simulink model "Flight_Controllers_PIL"  (R2024a)
settings: Solver=FixedStepAuto  StartTime=0.0  StopTime=tFinal  FixedStep=0.02  RelTol=1e-3  EnableMultiTasking=on
values from neighbouring files (symbols this model uses):
  bOmega = -bThrust/mThrust    (= 168.963839792)    [Load_VehicleParams.m]
  Cant_cosine_Loss = cos(fanCantAngle)    [Load_VehicleParams.m]
  g = 9.807    [Load_VehicleParams.m]
  g_Offset = 5/6    (= 0.833333333333)    [Load_VehicleParams.m]
  Kd_LatPos = 0    [Load_Controller_Gains_14.m]
  Kd_LatVel = 0    [Load_Controller_Gains_14.m]
  Kd_Pitch = 41.5    [Load_Controller_Gains_14.m]
  Ki_LatPos = 0    [Load_Controller_Gains_14.m]
  Ki_LatVel = 0    [Load_Controller_Gains_14.m]
  Ki_Pitch = 0.65    [Load_Controller_Gains_14.m]
  Kp_LatPos = 0.4    [Load_Controller_Gains_14.m]
  Kp_LatVel = -0.3    [Load_Controller_Gains_14.m]
  Kp_Pitch = 16    [Load_Controller_Gains_14.m]
  mOmega = 1/mThrust    (= 1.62153397114)    [Load_VehicleParams.m]
  N_LatPos = 0    [Load_Controller_Gains_14.m]
  N_LatVel = 0    [Load_Controller_Gains_14.m]
  N_Pitch = 85.6    [Load_Controller_Gains_14.m]
  nFans = 4    [Load_VehicleParams.m]
  pitch_Cmd_Limit = 7*pi/180    (= 0.12217304764)    [Load_Controller_Gains_14.m]
  T = 0.02    [run_Lander_GNC_Sim.m]
  tau_vCmd = 0.1    [Load_Controller_Gains_14.m]
  Ts_Control = 1/50    (= 0.02)    [run_Lander_GNC_Sim.m]
  velCmd_Limit = 7*pi/180    (= 0.12217304764)    [Load_Controller_Gains_14.m]
undefined symbols (not defined in the file or in its folder): den_Gc_z_Pitch, den_Gc_z_Pos, DiscIntNeverNeededParam, num_Gc_z_Pitch, num_Gc_z_Pos, posCntrl_Integr_Limit, tau_LatPos, tau_xCmd, vCmd_Integr_Limit
libraries: slpidlib x17
(part 2 of 3)

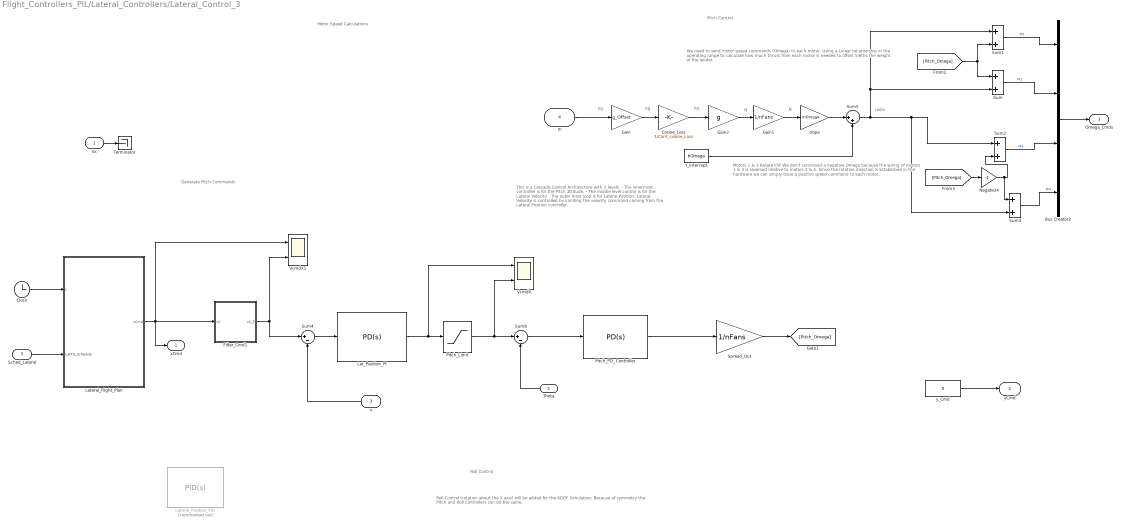
== system Flight_Controllers_PIL/Lateral_Controllers/Lateral_Control_3 ==
  note: Roll Control (rotation about the X axis) will be added for the 6DOF Simulation. Because of symmetry the Pitch and Roll Controllers can be the same.
  note: N
  note: Motors 1 & 3 Rotate CW
      | We don't command a negative Omega because the
      | wiring of motors 1 & 3 is reversed relative to motors 2 & 4.
      |
      | Since the rotation direction is established in the hardware
      | we can simply issue a positive speed command to each motor.
  note: We need to send motor speed commands (Omega) to each motor.
      |
      | Using a Linear rel;ationship in the operating range to calculate how much thrust from each motor is needed to offset 5/6ths the weight of the lander.
  note: Motor Speed Calculations
  note: kg
  note: kg
  note: N
  note: kg
  note: rad/s
  note: Pitch Control
  note: Roll Control
  note: Generate Pitch Commands
  note: This is a Cascade Control Architecture with 3 levels.
      | - The innermost controller is for the Pitch attitude.
      | - The middle level control is for the Lateral Velocity
      | - The outer most loop is for Lateral Position.
      | Lateral Velocity is controlled by Limiting the velocity command coming from the Lateral Position controller.
  Vx : Inport
  Theta : Inport  Port=2
  x : Inport  Port=3
  m : Inport  Port=4
  Sched_Lateral : Inport  Port=5
  Bus Creator2 : BusCreator  Inputs=4  OutDataTypeStr=Bus: MotorCmd_Bus
  Clock : Clock
  Cosine_Loss : Gain  Gain=1/Cant_cosine_Loss
  Filter_Cmd1 : Subsystem
  Gain : Gain  Gain=g_Offset
  Gain1 : Gain  Gain=1/nFans
  Gain2 : Gain  Gain=g
  Lat_Position_PI : slpidlib/PID Controller  Controller=PD  Form=Parallel  TimeDomain=Continuous-time  UseExternalTs=off  SampleTime=-1  IntegratorMethod=Forward Euler  FilterMethod=Forward Euler  ControllerParametersSource=internal  P=Kp_LatPos  I=-0.1  UseKiTs=off  D=Kd_LatPos  UseExternalDerivativeSource=off  N=N_LatPos  UseFilter=on  TunerSelectOption=Transfer Function Based (PID Tuner App)  InitialConditionSource=internal  InitialConditionForIntegrator=0  InitialConditionForFilter=0  DifferentiatorICPrevScaledInput=0  ExternalReset=none  TrackingMode=off  Kt=1  LimitOutput=off  SatLimitsSource=internal  UpperSaturationLimit=inf  LowerSaturationLimit=-inf  LinearizeAsGain=on  AntiWindupMode=none  Kb=1  LimitIntegrator=off  UpperIntegratorSaturationLimit=posCntrl_Integr_Limit  LowerIntegratorSaturationLimit=-posCntrl_Integr_Limit  POutMin=[]  POutMax=[]  IOutMin=[]  IOutMax=[]  DOutMin=[]  DOutMax=[]  NOutMin=[]  NOutMax=[]  SumOutMin=[]  SumOutMax=[]  SaturationOutMin=[]  SaturationOutMax=[]  PParamMin=[]  PParamMax=[]  IParamMin=[]  IParamMax=[]  DParamMin=[]  DParamMax=[]  NParamMin=[]  NParamMax=[]  KbParamMin=[]  KbParamMax=[]  KtParamMin=[]  KtParamMax=[]  KbOutMin=[]  KbOutMax=[]  KtOutMin=[]  KtOutMax=[]  IntegratorOutMin=[]  IntegratorOutMax=[]  FilterOutMin=[]  FilterOutMax=[]  SumI1OutMin=[]  SumI1OutMax=[]  SumI2OutMin=[]  SumI2OutMax=[]  SumI3OutMin=[]  SumI3OutMax=[]  SumI4OutMin=[]  SumI4OutMax=[]  SumDOutMin=[]  SumDOutMax=[]  DifferentiatorOutMin=[]  DifferentiatorOutMax=[]  FilterDiffOutCoefMin=[]  FilterDiffOutCoefMax=[]  ReciprocalOutMin=[]  ReciprocalOutMax=[]  SumDenOutMin=[]  SumDenOutMax=[]  SumNumOutMin=[]  SumNumOutMax=[]  DivideOutMin=[]  DivideOutMax=[]  UdiffTsProdOutMin=[]  UdiffTsProdOutMax=[]  NTsProdOutMin=[]  NTsProdOutMax=[]  UintegralTsProdOutMin=[]  UintegralTsProdOutMax=[]  UngainTsProdOutMin=[]  UngainTsProdOutMax=[]  ClampingZeroOutDataTypeStr=Inherit: Inherit via back propagation  ClampingZeroOutMin=[]  ClampingZeroOutMax=[]  FilterDenConstantOutDataTypeStr=Inherit: Inherit via back propagation  FilterDenConstantOutMin=[]  FilterDenConstantOutMax=[]  PCopyOutDataTypeStr=Inherit: Inherit via back propagation  PCopyOutMin=[]  PCopyOutMax=[]  NCopyOutDataTypeStr=Inherit: Inherit via back propagation  NCopyOutMin=[]  NCopyOutMax=[]  IntegratorContinuousStateAttributes=''  IntegratorStateMustResolveToSignalObject=off  IntegratorRTWStateStorageClass=Auto  FilterContinuousStateAttributes=''  FilterStateMustResolveToSignalObject=off  FilterRTWStateStorageClass=Auto  ParallelPVariant=InternalParameters  IdealPVariant=Disabled  IVariant=Disabled  DVariant=InternalParameters  IntegratorVariant=Disabled  SatVariant=Disabled  AWVariant=Disabled  PCopyVariant=Disabled  TRVariant=Disabled  FdbkBlocksVariant=Forward  IdealPFdbkVariant=Disabled  SatFdbkVariant=Disabled  DerivativeFilterVariant=ContFilter  NVariant=InternalParameters  NCopyVariant=Disabled  FilterICVariant=InternalICsFilter  IntegratorICVariant=Disabled  ExternalResetVariant=Disabled  TRSumVariant=Passthrough  SumFdbkVariant=Disabled  SumVariant=Sum_PD  TsampFilterVariant=InternalTs  TsampNgainVariant=Passthrough  TsampIntegralVariant=Disabled_SignalSpec  ExternalSaturationOutDataTypeStr=Inherit: Same as second input  DerivativeSourceVariant=ErrorSignal
  Lateral_Flight_Plan : MATLAB Function  TreatAsAtomicUnit=on
  Lateral_Position_PID : slpidlib/PID Controller  Commented=on  Controller=PID  Form=Parallel  TimeDomain=Continuous-time  UseExternalTs=off  SampleTime=-1  IntegratorMethod=Forward Euler  FilterMethod=Forward Euler  ControllerParametersSource=internal  P=Kp_LatPos  I=Ki_LatPos  UseKiTs=off  D=Kd_LatPos  UseExternalDerivativeSource=off  N=N_LatPos  UseFilter=on  TunerSelectOption=Transfer Function Based (PID Tuner App)  InitialConditionSource=internal  InitialConditionForIntegrator=0  InitialConditionForFilter=0  DifferentiatorICPrevScaledInput=0  ExternalReset=none  TrackingMode=off  Kt=1  LimitOutput=off  SatLimitsSource=internal  UpperSaturationLimit=inf  LowerSaturationLimit=-inf  LinearizeAsGain=on  AntiWindupMode=none  Kb=1  LimitIntegrator=on  UpperIntegratorSaturationLimit=vCmd_Integr_Limit  LowerIntegratorSaturationLimit=-vCmd_Integr_Limit  POutMin=[]  POutMax=[]  IOutMin=[]  IOutMax=[]  DOutMin=[]  DOutMax=[]  NOutMin=[]  NOutMax=[]  SumOutMin=[]  SumOutMax=[]  SaturationOutMin=[]  SaturationOutMax=[]  PParamMin=[]  PParamMax=[]  IParamMin=[]  IParamMax=[]  DParamMin=[]  DParamMax=[]  NParamMin=[]  NParamMax=[]  KbParamMin=[]  KbParamMax=[]  KtParamMin=[]  KtParamMax=[]  KbOutMin=[]  KbOutMax=[]  KtOutMin=[]  KtOutMax=[]  IntegratorOutMin=[]  IntegratorOutMax=[]  FilterOutMin=[]  FilterOutMax=[]  SumI1OutMin=[]  SumI1OutMax=[]  SumI2OutMin=[]  SumI2OutMax=[]  SumI3OutMin=[]  SumI3OutMax=[]  SumI4OutMin=[]  SumI4OutMax=[]  SumDOutMin=[]  SumDOutMax=[]  DifferentiatorOutMin=[]  DifferentiatorOutMax=[]  FilterDiffOutCoefMin=[]  FilterDiffOutCoefMax=[]  ReciprocalOutMin=[]  ReciprocalOutMax=[]  SumDenOutMin=[]  SumDenOutMax=[]  SumNumOutMin=[]  SumNumOutMax=[]  DivideOutMin=[]  DivideOutMax=[]  UdiffTsProdOutMin=[]  UdiffTsProdOutMax=[]  NTsProdOutMin=[]  NTsProdOutMax=[]  UintegralTsProdOutMin=[]  UintegralTsProdOutMax=[]  UngainTsProdOutMin=[]  UngainTsProdOutMax=[]  ClampingZeroOutDataTypeStr=Inherit: Inherit via back propagation  ClampingZeroOutMin=[]  ClampingZeroOutMax=[]  FilterDenConstantOutDataTypeStr=Inherit: Inherit via back propagation  FilterDenConstantOutMin=[]  FilterDenConstantOutMax=[]  PCopyOutDataTypeStr=Inherit: Inherit via back propagation  PCopyOutMin=[]  PCopyOutMax=[]  NCopyOutDataTypeStr=Inherit: Inherit via back propagation  NCopyOutMin=[]  NCopyOutMax=[]  IntegratorContinuousStateAttributes=''  IntegratorStateMustResolveToSignalObject=off  IntegratorRTWStateStorageClass=Auto  FilterContinuousStateAttributes=''  FilterStateMustResolveToSignalObject=off  FilterRTWStateStorageClass=Auto  ParallelPVariant=InternalParameters  IdealPVariant=Disabled  IVariant=InternalParameters  DVariant=InternalParameters  IntegratorVariant=Continuous  SatVariant=Disabled  AWVariant=Passthrough  PCopyVariant=Disabled  TRVariant=Disabled  FdbkBlocksVariant=Forward  IdealPFdbkVariant=Disabled  SatFdbkVariant=Disabled  DerivativeFilterVariant=ContFilter  NVariant=InternalParameters  NCopyVariant=Disabled  FilterICVariant=InternalICsFilter  IntegratorICVariant=InternalICs  ExternalResetVariant=Disabled  TRSumVariant=Passthrough  SumFdbkVariant=Disabled  SumVariant=Sum_PID  TsampFilterVariant=InternalTs  TsampNgainVariant=Passthrough  TsampIntegralVariant=Disabled_SignalSpec  ExternalSaturationOutDataTypeStr=Inherit: Same as second input  DerivativeSourceVariant=ErrorSignal
  Negate34 : Gain  Gain=-1
  Pitch_Limit : Saturate  UpperLimit=pitch_Cmd_Limit  LowerLimit=-pitch_Cmd_Limit
  Pitch_PD_ Controller : slpidlib/PID Controller  Controller=PD  Form=Parallel  TimeDomain=Continuous-time  UseExternalTs=off  SampleTime=-1  IntegratorMethod=Forward Euler  FilterMethod=Forward Euler  ControllerParametersSource=internal  P=Kp_Pitch  I=1  UseKiTs=off  D=Kd_Pitch  UseExternalDerivativeSource=off  N=N_Pitch  UseFilter=on  TunerSelectOption=Transfer Function Based (PID Tuner App)  InitialConditionSource=internal  InitialConditionForIntegrator=0  InitialConditionForFilter=0  DifferentiatorICPrevScaledInput=0  ExternalReset=none  TrackingMode=off  Kt=1  LimitOutput=off  SatLimitsSource=internal  UpperSaturationLimit=inf  LowerSaturationLimit=-inf  LinearizeAsGain=on  AntiWindupMode=none  Kb=1  LimitIntegrator=off  UpperIntegratorSaturationLimit=inf  LowerIntegratorSaturationLimit=-inf  POutMin=[]  POutMax=[]  IOutMin=[]  IOutMax=[]  DOutMin=[]  DOutMax=[]  NOutMin=[]  NOutMax=[]  SumOutMin=[]  SumOutMax=[]  SaturationOutMin=[]  SaturationOutMax=[]  PParamMin=[]  PParamMax=[]  IParamMin=[]  IParamMax=[]  DParamMin=[]  DParamMax=[]  NParamMin=[]  NParamMax=[]  KbParamMin=[]  KbParamMax=[]  KtParamMin=[]  KtParamMax=[]  KbOutMin=[]  KbOutMax=[]  KtOutMin=[]  KtOutMax=[]  IntegratorOutMin=[]  IntegratorOutMax=[]  FilterOutMin=[]  FilterOutMax=[]  SumI1OutMin=[]  SumI1OutMax=[]  SumI2OutMin=[]  SumI2OutMax=[]  SumI3OutMin=[]  SumI3OutMax=[]  SumI4OutMin=[]  SumI4OutMax=[]  SumDOutMin=[]  SumDOutMax=[]  DifferentiatorOutMin=[]  DifferentiatorOutMax=[]  FilterDiffOutCoefMin=[]  FilterDiffOutCoefMax=[]  ReciprocalOutMin=[]  ReciprocalOutMax=[]  SumDenOutMin=[]  SumDenOutMax=[]  SumNumOutMin=[]  SumNumOutMax=[]  DivideOutMin=[]  DivideOutMax=[]  UdiffTsProdOutMin=[]  UdiffTsProdOutMax=[]  NTsProdOutMin=[]  NTsProdOutMax=[]  UintegralTsProdOutMin=[]  UintegralTsProdOutMax=[]  UngainTsProdOutMin=[]  UngainTsProdOutMax=[]  ClampingZeroOutDataTypeStr=Inherit: Inherit via back propagation  ClampingZeroOutMin=[]  ClampingZeroOutMax=[]  FilterDenConstantOutDataTypeStr=Inherit: Inherit via back propagation  FilterDenConstantOutMin=[]  FilterDenConstantOutMax=[]  PCopyOutDataTypeStr=Inherit: Inherit via back propagation  PCopyOutMin=[]  PCopyOutMax=[]  NCopyOutDataTypeStr=Inherit: Inherit via back propagation  NCopyOutMin=[]  NCopyOutMax=[]  IntegratorContinuousStateAttributes=''  IntegratorStateMustResolveToSignalObject=off  IntegratorRTWStateStorageClass=Auto  FilterContinuousStateAttributes=''  FilterStateMustResolveToSignalObject=off  FilterRTWStateStorageClass=Auto  ParallelPVariant=InternalParameters  IdealPVariant=Disabled  IVariant=Disabled  DVariant=InternalParameters  IntegratorVariant=Disabled  SatVariant=Disabled  AWVariant=Disabled  PCopyVariant=Disabled  TRVariant=Disabled  FdbkBlocksVariant=Forward  IdealPFdbkVariant=Disabled  SatFdbkVariant=Disabled  DerivativeFilterVariant=ContFilter  NVariant=InternalParameters  NCopyVariant=Disabled  FilterICVariant=InternalICsFilter  IntegratorICVariant=Disabled  ExternalResetVariant=Disabled  TRSumVariant=Passthrough  SumFdbkVariant=Disabled  SumVariant=Sum_PD  TsampFilterVariant=InternalTs  TsampNgainVariant=Passthrough  TsampIntegralVariant=Disabled_SignalSpec  ExternalSaturationOutDataTypeStr=Inherit: Same as second input  DerivativeSourceVariant=ErrorSignal
  Spread_Out : Gain  Gain=1/nFans
  Sum{,1..3} (4 alike) : Sum
  Sum4 : Sum  Inputs=|+-
  Sum5 : Sum  Inputs=|++
  Sum8 : Sum  Inputs=|+-
  Terminator : Terminator
  VcmdX : Scope  NumInputPorts=2
  VcmdX1 : Scope  NumInputPorts=2
  Y_intercept : Constant  Value=bOmega
  slope : Gain  Gain=mOmega
  y_Cmd : Constant  Value=0
  xCmd : Outport
  yCmd : Outport  Port=2
  Omega_Cmds : Outport  Port=3
  wires:
  Clock/1 -> Lateral_Flight_Plan/1(t)
  Lateral_Flight_Plan/1(xCmd) -> Filter_Cmd1/1(xC), xCmd/1, VcmdX1/1
  Gain2/1 -> Gain1/1
  Sum3/1 -> Bus Creator2/4  "M4"
  Negate34/1 -> Sum3/1, Sum2/2
  Gain1/1 -> slope/1
  Bus Creator2/1 -> Omega_Cmds/1
  slope/1 -> Sum5/1
  Sum1/1 -> Bus Creator2/1  "M1"
  Sum5/1 -> Sum3/2, Sum2/1, Sum1/1, Sum/2
  Y_intercept/1 -> Sum5/2
  Sum/1 -> Bus Creator2/2  "M2"
  m/1 -> Gain/1
  Cosine_Loss/1 -> Gain2/1
  Gain/1 -> Cosine_Loss/1
  Spread_Out/1 -> [Pitch_Omega]
  [Pitch_Omega] -> Sum/1, Sum1/2
  Sum2/1 -> Bus Creator2/3  "M3"
  [Pitch_Omega] -> Negate34/1
  Sched_Lateral/1 -> Lateral_Flight_Plan/2(LatFlt_Schedule)
  Pitch_PD_ Controller/1 -> Spread_Out/1
  Filter_Cmd1/1(xC_F) -> Sum4/1, VcmdX1/2
  x/1 -> Sum4/2
  Vx/1 -> Terminator/1
  Theta/1 -> Sum8/2
  Lat_Position_PI/1 -> VcmdX/1, Pitch_Limit/1
  Pitch_Limit/1 -> VcmdX/2, Sum8/1
  Sum8/1 -> Pitch_PD_ Controller/1
  Sum4/1 -> Lat_Position_PI/1
  y_Cmd/1 -> yCmd/1

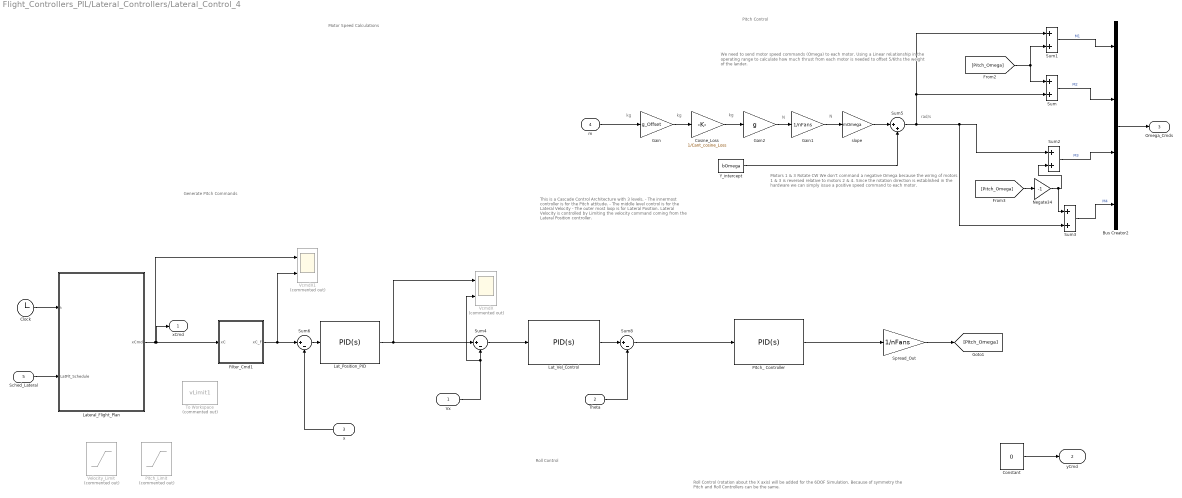
== system Flight_Controllers_PIL/Lateral_Controllers/Lateral_Control_4 ==
  note: kg
  note: kg
  note: N
  note: Motor Speed Calculations
  note: We need to send motor speed commands (Omega) to each motor.
      |
      | Using a Linear rel;ationship in the operating range to calculate how much thrust from each motor is needed to offset 5/6ths the weight of the lander.
  note: Motors 1 & 3 Rotate CW
      | We don't command a negative Omega because the
      | wiring of motors 1 & 3 is reversed relative to motors 2 & 4.
      |
      | Since the rotation direction is established in the hardware
      | we can simply issue a positive speed command to each motor.
  note: Roll Control (rotation about the X axis) will be added for the 6DOF Simulation. Because of symmetry the Pitch and Roll Controllers can be the same.
  note: N
  note: kg
  note: Roll Control
  note: rad/s
  note: Generate Pitch Commands
  note: This is a Cascade Control Architecture with 3 levels.
      | - The innermost controller is for the Pitch attitude.
      | - The middle level control is for the Lateral Velocity
      | - The outer most loop is for Lateral Position.
      | Lateral Velocity is controlled by Limiting the velocity command coming from the Lateral Position controller.
  note: Pitch Control
  Vx : Inport
  Theta : Inport  Port=2
  x : Inport  Port=3
  m : Inport  Port=4
  Sched_Lateral : Inport  Port=5
  Bus Creator2 : BusCreator  Inputs=4  OutDataTypeStr=Bus: MotorCmd_Bus
  Clock : Clock
  Constant : Constant  Value=0
  Cosine_Loss : Gain  Gain=1/Cant_cosine_Loss
  Filter_Cmd1 : Subsystem
  Gain : Gain  Gain=g_Offset
  Gain1 : Gain  Gain=1/nFans
  Gain2 : Gain  Gain=g
  Lat_Position_PID : slpidlib/PID Controller  Controller=PID  Form=Parallel  TimeDomain=Continuous-time  UseExternalTs=off  SampleTime=-1  IntegratorMethod=Forward Euler  FilterMethod=Forward Euler  ControllerParametersSource=internal  P=Kp_LatPos  I=Ki_LatPos  UseKiTs=off  D=Kd_LatPos  UseExternalDerivativeSource=off  N=N_LatPos  UseFilter=on  TunerSelectOption=Transfer Function Based (PID Tuner App)  InitialConditionSource=internal  InitialConditionForIntegrator=0  InitialConditionForFilter=0  DifferentiatorICPrevScaledInput=0  ExternalReset=none  TrackingMode=off  Kt=1  LimitOutput=off  SatLimitsSource=internal  UpperSaturationLimit=inf  LowerSaturationLimit=-inf  LinearizeAsGain=on  AntiWindupMode=none  Kb=1  LimitIntegrator=off  UpperIntegratorSaturationLimit=vCmd_Integr_Limit  LowerIntegratorSaturationLimit=-vCmd_Integr_Limit  POutMin=[]  POutMax=[]  IOutMin=[]  IOutMax=[]  DOutMin=[]  DOutMax=[]  NOutMin=[]  NOutMax=[]  SumOutMin=[]  SumOutMax=[]  SaturationOutMin=[]  SaturationOutMax=[]  PParamMin=[]  PParamMax=[]  IParamMin=[]  IParamMax=[]  DParamMin=[]  DParamMax=[]  NParamMin=[]  NParamMax=[]  KbParamMin=[]  KbParamMax=[]  KtParamMin=[]  KtParamMax=[]  KbOutMin=[]  KbOutMax=[]  KtOutMin=[]  KtOutMax=[]  IntegratorOutMin=[]  IntegratorOutMax=[]  FilterOutMin=[]  FilterOutMax=[]  SumI1OutMin=[]  SumI1OutMax=[]  SumI2OutMin=[]  SumI2OutMax=[]  SumI3OutMin=[]  SumI3OutMax=[]  SumI4OutMin=[]  SumI4OutMax=[]  SumDOutMin=[]  SumDOutMax=[]  DifferentiatorOutMin=[]  DifferentiatorOutMax=[]  FilterDiffOutCoefMin=[]  FilterDiffOutCoefMax=[]  ReciprocalOutMin=[]  ReciprocalOutMax=[]  SumDenOutMin=[]  SumDenOutMax=[]  SumNumOutMin=[]  SumNumOutMax=[]  DivideOutMin=[]  DivideOutMax=[]  UdiffTsProdOutMin=[]  UdiffTsProdOutMax=[]  NTsProdOutMin=[]  NTsProdOutMax=[]  UintegralTsProdOutMin=[]  UintegralTsProdOutMax=[]  UngainTsProdOutMin=[]  UngainTsProdOutMax=[]  ClampingZeroOutDataTypeStr=Inherit: Inherit via back propagation  ClampingZeroOutMin=[]  ClampingZeroOutMax=[]  FilterDenConstantOutDataTypeStr=Inherit: Inherit via back propagation  FilterDenConstantOutMin=[]  FilterDenConstantOutMax=[]  PCopyOutDataTypeStr=Inherit: Inherit via back propagation  PCopyOutMin=[]  PCopyOutMax=[]  NCopyOutDataTypeStr=Inherit: Inherit via back propagation  NCopyOutMin=[]  NCopyOutMax=[]  IntegratorContinuousStateAttributes=''  IntegratorStateMustResolveToSignalObject=off  IntegratorRTWStateStorageClass=Auto  FilterContinuousStateAttributes=''  FilterStateMustResolveToSignalObject=off  FilterRTWStateStorageClass=Auto  ParallelPVariant=InternalParameters  IdealPVariant=Disabled  IVariant=InternalParameters  DVariant=InternalParameters  IntegratorVariant=Continuous  SatVariant=Disabled  AWVariant=Passthrough  PCopyVariant=Disabled  TRVariant=Disabled  FdbkBlocksVariant=Forward  IdealPFdbkVariant=Disabled  SatFdbkVariant=Disabled  DerivativeFilterVariant=ContFilter  NVariant=InternalParameters  NCopyVariant=Disabled  FilterICVariant=InternalICsFilter  IntegratorICVariant=InternalICs  ExternalResetVariant=Disabled  TRSumVariant=Passthrough  SumFdbkVariant=Disabled  SumVariant=Sum_PID  TsampFilterVariant=InternalTs  TsampNgainVariant=Passthrough  TsampIntegralVariant=Disabled_SignalSpec  ExternalSaturationOutDataTypeStr=Inherit: Same as second input  DerivativeSourceVariant=ErrorSignal
  Lat_Vel_Control : slpidlib/PID Controller  Controller=PID  Form=Parallel  TimeDomain=Continuous-time  UseExternalTs=off  SampleTime=-1  IntegratorMethod=Forward Euler  FilterMethod=Forward Euler  ControllerParametersSource=internal  P=Kp_LatVel  I=Ki_LatVel  UseKiTs=off  D=Kd_LatVel  UseExternalDerivativeSource=off  N=N_LatVel  UseFilter=on  TunerSelectOption=Transfer Function Based (PID Tuner App)  InitialConditionSource=internal  InitialConditionForIntegrator=0  InitialConditionForFilter=0  DifferentiatorICPrevScaledInput=0  ExternalReset=none  TrackingMode=off  Kt=1  LimitOutput=off  SatLimitsSource=internal  UpperSaturationLimit=inf  LowerSaturationLimit=-inf  LinearizeAsGain=on  AntiWindupMode=none  Kb=1  LimitIntegrator=off  UpperIntegratorSaturationLimit=inf  LowerIntegratorSaturationLimit=-inf  POutMin=[]  POutMax=[]  IOutMin=[]  IOutMax=[]  DOutMin=[]  DOutMax=[]  NOutMin=[]  NOutMax=[]  SumOutMin=[]  SumOutMax=[]  SaturationOutMin=[]  SaturationOutMax=[]  PParamMin=[]  PParamMax=[]  IParamMin=[]  IParamMax=[]  DParamMin=[]  DParamMax=[]  NParamMin=[]  NParamMax=[]  KbParamMin=[]  KbParamMax=[]  KtParamMin=[]  KtParamMax=[]  KbOutMin=[]  KbOutMax=[]  KtOutMin=[]  KtOutMax=[]  IntegratorOutMin=[]  IntegratorOutMax=[]  FilterOutMin=[]  FilterOutMax=[]  SumI1OutMin=[]  SumI1OutMax=[]  SumI2OutMin=[]  SumI2OutMax=[]  SumI3OutMin=[]  SumI3OutMax=[]  SumI4OutMin=[]  SumI4OutMax=[]  SumDOutMin=[]  SumDOutMax=[]  DifferentiatorOutMin=[]  DifferentiatorOutMax=[]  FilterDiffOutCoefMin=[]  FilterDiffOutCoefMax=[]  ReciprocalOutMin=[]  ReciprocalOutMax=[]  SumDenOutMin=[]  SumDenOutMax=[]  SumNumOutMin=[]  SumNumOutMax=[]  DivideOutMin=[]  DivideOutMax=[]  UdiffTsProdOutMin=[]  UdiffTsProdOutMax=[]  NTsProdOutMin=[]  NTsProdOutMax=[]  UintegralTsProdOutMin=[]  UintegralTsProdOutMax=[]  UngainTsProdOutMin=[]  UngainTsProdOutMax=[]  ClampingZeroOutDataTypeStr=Inherit: Inherit via back propagation  ClampingZeroOutMin=[]  ClampingZeroOutMax=[]  FilterDenConstantOutDataTypeStr=Inherit: Inherit via back propagation  FilterDenConstantOutMin=[]  FilterDenConstantOutMax=[]  PCopyOutDataTypeStr=Inherit: Inherit via back propagation  PCopyOutMin=[]  PCopyOutMax=[]  NCopyOutDataTypeStr=Inherit: Inherit via back propagation  NCopyOutMin=[]  NCopyOutMax=[]  IntegratorContinuousStateAttributes=''  IntegratorStateMustResolveToSignalObject=off  IntegratorRTWStateStorageClass=Auto  FilterContinuousStateAttributes=''  FilterStateMustResolveToSignalObject=off  FilterRTWStateStorageClass=Auto  ParallelPVariant=InternalParameters  IdealPVariant=Disabled  IVariant=InternalParameters  DVariant=InternalParameters  IntegratorVariant=Continuous  SatVariant=Disabled  AWVariant=Passthrough  PCopyVariant=Disabled  TRVariant=Disabled  FdbkBlocksVariant=Forward  IdealPFdbkVariant=Disabled  SatFdbkVariant=Disabled  DerivativeFilterVariant=ContFilter  NVariant=InternalParameters  NCopyVariant=Disabled  FilterICVariant=InternalICsFilter  IntegratorICVariant=InternalICs  ExternalResetVariant=Disabled  TRSumVariant=Passthrough  SumFdbkVariant=Disabled  SumVariant=Sum_PID  TsampFilterVariant=InternalTs  TsampNgainVariant=Passthrough  TsampIntegralVariant=Disabled_SignalSpec  ExternalSaturationOutDataTypeStr=Inherit: Same as second input  DerivativeSourceVariant=ErrorSignal
  Lateral_Flight_Plan : MATLAB Function  TreatAsAtomicUnit=on
  Negate34 : Gain  Gain=-1
  Pitch_ Controller : slpidlib/PID Controller  Controller=PID  Form=Parallel  TimeDomain=Continuous-time  UseExternalTs=off  SampleTime=-1  IntegratorMethod=Forward Euler  FilterMethod=Forward Euler  ControllerParametersSource=internal  P=Kp_Pitch  I=Ki_Pitch  UseKiTs=off  D=Kd_Pitch  UseExternalDerivativeSource=off  N=N_Pitch  UseFilter=on  TunerSelectOption=Transfer Function Based (PID Tuner App)  InitialConditionSource=internal  InitialConditionForIntegrator=0  InitialConditionForFilter=0  DifferentiatorICPrevScaledInput=0  ExternalReset=none  TrackingMode=off  Kt=1  LimitOutput=off  SatLimitsSource=internal  UpperSaturationLimit=inf  LowerSaturationLimit=-inf  LinearizeAsGain=on  AntiWindupMode=none  Kb=1  LimitIntegrator=off  UpperIntegratorSaturationLimit=inf  LowerIntegratorSaturationLimit=-inf  POutMin=[]  POutMax=[]  IOutMin=[]  IOutMax=[]  DOutMin=[]  DOutMax=[]  NOutMin=[]  NOutMax=[]  SumOutMin=[]  SumOutMax=[]  SaturationOutMin=[]  SaturationOutMax=[]  PParamMin=[]  PParamMax=[]  IParamMin=[]  IParamMax=[]  DParamMin=[]  DParamMax=[]  NParamMin=[]  NParamMax=[]  KbParamMin=[]  KbParamMax=[]  KtParamMin=[]  KtParamMax=[]  KbOutMin=[]  KbOutMax=[]  KtOutMin=[]  KtOutMax=[]  IntegratorOutMin=[]  IntegratorOutMax=[]  FilterOutMin=[]  FilterOutMax=[]  SumI1OutMin=[]  SumI1OutMax=[]  SumI2OutMin=[]  SumI2OutMax=[]  SumI3OutMin=[]  SumI3OutMax=[]  SumI4OutMin=[]  SumI4OutMax=[]  SumDOutMin=[]  SumDOutMax=[]  DifferentiatorOutMin=[]  DifferentiatorOutMax=[]  FilterDiffOutCoefMin=[]  FilterDiffOutCoefMax=[]  ReciprocalOutMin=[]  ReciprocalOutMax=[]  SumDenOutMin=[]  SumDenOutMax=[]  SumNumOutMin=[]  SumNumOutMax=[]  DivideOutMin=[]  DivideOutMax=[]  UdiffTsProdOutMin=[]  UdiffTsProdOutMax=[]  NTsProdOutMin=[]  NTsProdOutMax=[]  UintegralTsProdOutMin=[]  UintegralTsProdOutMax=[]  UngainTsProdOutMin=[]  UngainTsProdOutMax=[]  ClampingZeroOutDataTypeStr=Inherit: Inherit via back propagation  ClampingZeroOutMin=[]  ClampingZeroOutMax=[]  FilterDenConstantOutDataTypeStr=Inherit: Inherit via back propagation  FilterDenConstantOutMin=[]  FilterDenConstantOutMax=[]  PCopyOutDataTypeStr=Inherit: Inherit via back propagation  PCopyOutMin=[]  PCopyOutMax=[]  NCopyOutDataTypeStr=Inherit: Inherit via back propagation  NCopyOutMin=[]  NCopyOutMax=[]  IntegratorContinuousStateAttributes=''  IntegratorStateMustResolveToSignalObject=off  IntegratorRTWStateStorageClass=Auto  FilterContinuousStateAttributes=''  FilterStateMustResolveToSignalObject=off  FilterRTWStateStorageClass=Auto  ParallelPVariant=InternalParameters  IdealPVariant=Disabled  IVariant=InternalParameters  DVariant=InternalParameters  IntegratorVariant=Continuous  SatVariant=Disabled  AWVariant=Passthrough  PCopyVariant=Disabled  TRVariant=Disabled  FdbkBlocksVariant=Forward  IdealPFdbkVariant=Disabled  SatFdbkVariant=Disabled  DerivativeFilterVariant=ContFilter  NVariant=InternalParameters  NCopyVariant=Disabled  FilterICVariant=InternalICsFilter  IntegratorICVariant=InternalICs  ExternalResetVariant=Disabled  TRSumVariant=Passthrough  SumFdbkVariant=Disabled  SumVariant=Sum_PID  TsampFilterVariant=InternalTs  TsampNgainVariant=Passthrough  TsampIntegralVariant=Disabled_SignalSpec  ExternalSaturationOutDataTypeStr=Inherit: Same as second input  DerivativeSourceVariant=ErrorSignal
  Pitch_Limit : Saturate  Commented=on  UpperLimit=pitch_Cmd_Limit  LowerLimit=-pitch_Cmd_Limit
  Spread_Out : Gain  Gain=1/nFans
  Sum{,1..3} (4 alike) : Sum
  Sum4 : Sum  Inputs=|+-
  Sum5 : Sum  Inputs=|++
  Sum6 : Sum  Inputs=|+-
  Sum8 : Sum  Inputs=|+-
  To Workspace : ToWorkspace  Commented=on  VariableName=vLimit1  SaveFormat=Timeseries  SampleTime=-1
  VcmdX : Scope  Commented=on  NumInputPorts=2
  VcmdX1 : Scope  Commented=on  NumInputPorts=2
  Velocity_Limit : Saturate  Commented=on  UpperLimit=velCmd_Limit  LowerLimit=-velCmd_Limit
  Y_intercept : Constant  Value=bOmega
  slope : Gain  Gain=mOmega
  xCmd : Outport
  yCmd : Outport  Port=2
  Omega_Cmds : Outport  Port=3
  wires:
  Sum8/1 -> Pitch_ Controller/1
  Sum/1 -> Bus Creator2/2  "M2"
  m/1 -> Gain/1
  Sched_Lateral/1 -> Lateral_Flight_Plan/2(LatFlt_Schedule)
  Constant/1 -> yCmd/1
  Filter_Cmd1/1(xC_F) -> VcmdX1/2, Sum6/1
  Bus Creator2/1 -> Omega_Cmds/1
  Clock/1 -> Lateral_Flight_Plan/1(t)
  Pitch_ Controller/1 -> Spread_Out/1
  x/1 -> Sum6/2
  Spread_Out/1 -> [Pitch_Omega]
  Lat_Position_PID/1 -> Sum4/1, VcmdX/1
  [Pitch_Omega] -> Sum/1, Sum1/2
  Sum1/1 -> Bus Creator2/1  "M1"
  Vx/1 -> VcmdX/2, Sum4/2
  Y_intercept/1 -> Sum5/2
  Negate34/1 -> Sum3/1, Sum2/2
  Sum5/1 -> Sum3/2, Sum2/1, Sum1/1, Sum/2
  Theta/1 -> Sum8/2
  slope/1 -> Sum5/1
  Lat_Vel_Control/1 -> Sum8/1
  Sum4/1 -> Lat_Vel_Control/1
  [Pitch_Omega] -> Negate34/1
  Gain/1 -> Cosine_Loss/1
  Cosine_Loss/1 -> Gain2/1
  Sum2/1 -> Bus Creator2/3  "M3"
  Gain1/1 -> slope/1
  Gain2/1 -> Gain1/1
  Lateral_Flight_Plan/1(xCmd) -> Filter_Cmd1/1(xC), xCmd/1, VcmdX1/1
  Sum3/1 -> Bus Creator2/4  "M4"
  Sum6/1 -> Lat_Position_PID/1

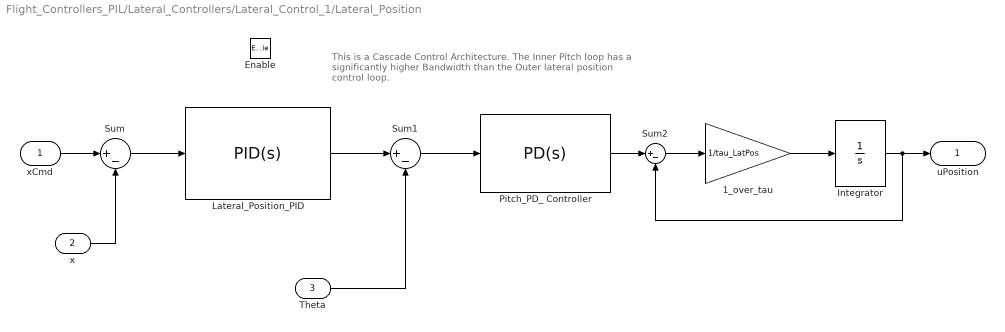
== system Flight_Controllers_PIL/Lateral_Controllers/Lateral_Control_1/Lateral_Position ==
  note: This is a Cascade Control Architecture.
      | The Inner Pitch loop has a significantly higher Bandwidth than
      | the Outer lateral position control loop.
  xCmd : Inport
  x : Inport  Port=2
  Theta : Inport  Port=3
  Enable : EnablePort
  1_over_tau : Gain  Gain=1/tau_LatPos
  Integrator : Integrator
  Lateral_Position_PID : slpidlib/PID Controller  Controller=PID  Form=Parallel  TimeDomain=Continuous-time  UseExternalTs=off  SampleTime=-1  IntegratorMethod=Forward Euler  FilterMethod=Forward Euler  ControllerParametersSource=internal  P=Kp_LatPos  I=Ki_LatPos  UseKiTs=off  D=Kd_LatPos  UseExternalDerivativeSource=off  N=N_LatPos  UseFilter=on  TunerSelectOption=Transfer Function Based (PID Tuner App)  InitialConditionSource=internal  InitialConditionForIntegrator=0  InitialConditionForFilter=0  DifferentiatorICPrevScaledInput=0  ExternalReset=none  TrackingMode=off  Kt=1  LimitOutput=off  SatLimitsSource=internal  UpperSaturationLimit=inf  LowerSaturationLimit=-inf  LinearizeAsGain=on  AntiWindupMode=none  Kb=1  LimitIntegrator=off  UpperIntegratorSaturationLimit=inf  LowerIntegratorSaturationLimit=-inf  POutMin=[]  POutMax=[]  IOutMin=[]  IOutMax=[]  DOutMin=[]  DOutMax=[]  NOutMin=[]  NOutMax=[]  SumOutMin=[]  SumOutMax=[]  SaturationOutMin=[]  SaturationOutMax=[]  PParamMin=[]  PParamMax=[]  IParamMin=[]  IParamMax=[]  DParamMin=[]  DParamMax=[]  NParamMin=[]  NParamMax=[]  KbParamMin=[]  KbParamMax=[]  KtParamMin=[]  KtParamMax=[]  KbOutMin=[]  KbOutMax=[]  KtOutMin=[]  KtOutMax=[]  IntegratorOutMin=[]  IntegratorOutMax=[]  FilterOutMin=[]  FilterOutMax=[]  SumI1OutMin=[]  SumI1OutMax=[]  SumI2OutMin=[]  SumI2OutMax=[]  SumI3OutMin=[]  SumI3OutMax=[]  SumI4OutMin=[]  SumI4OutMax=[]  SumDOutMin=[]  SumDOutMax=[]  DifferentiatorOutMin=[]  DifferentiatorOutMax=[]  FilterDiffOutCoefMin=[]  FilterDiffOutCoefMax=[]  ReciprocalOutMin=[]  ReciprocalOutMax=[]  SumDenOutMin=[]  SumDenOutMax=[]  SumNumOutMin=[]  SumNumOutMax=[]  DivideOutMin=[]  DivideOutMax=[]  UdiffTsProdOutMin=[]  UdiffTsProdOutMax=[]  NTsProdOutMin=[]  NTsProdOutMax=[]  UintegralTsProdOutMin=[]  UintegralTsProdOutMax=[]  UngainTsProdOutMin=[]  UngainTsProdOutMax=[]  ClampingZeroOutDataTypeStr=Inherit: Inherit via back propagation  ClampingZeroOutMin=[]  ClampingZeroOutMax=[]  FilterDenConstantOutDataTypeStr=Inherit: Inherit via back propagation  FilterDenConstantOutMin=[]  FilterDenConstantOutMax=[]  PCopyOutDataTypeStr=Inherit: Inherit via back propagation  PCopyOutMin=[]  PCopyOutMax=[]  NCopyOutDataTypeStr=Inherit: Inherit via back propagation  NCopyOutMin=[]  NCopyOutMax=[]  IntegratorContinuousStateAttributes=''  IntegratorStateMustResolveToSignalObject=off  IntegratorRTWStateStorageClass=Auto  FilterContinuousStateAttributes=''  FilterStateMustResolveToSignalObject=off  FilterRTWStateStorageClass=Auto  ParallelPVariant=InternalParameters  IdealPVariant=Disabled  IVariant=InternalParameters  DVariant=InternalParameters  IntegratorVariant=Continuous  SatVariant=Disabled  AWVariant=Passthrough  PCopyVariant=Disabled  TRVariant=Disabled  FdbkBlocksVariant=Forward  IdealPFdbkVariant=Disabled  SatFdbkVariant=Disabled  DerivativeFilterVariant=ContFilter  NVariant=InternalParameters  NCopyVariant=Disabled  FilterICVariant=InternalICsFilter  IntegratorICVariant=InternalICs  ExternalResetVariant=Disabled  TRSumVariant=Passthrough  SumFdbkVariant=Disabled  SumVariant=Sum_PID  TsampFilterVariant=InternalTs  TsampNgainVariant=Passthrough  TsampIntegralVariant=Disabled_SignalSpec  ExternalSaturationOutDataTypeStr=Inherit: Same as second input  DerivativeSourceVariant=ErrorSignal
  Pitch_PD_ Controller : slpidlib/PID Controller  Controller=PD  Form=Parallel  TimeDomain=Continuous-time  UseExternalTs=off  SampleTime=-1  IntegratorMethod=Forward Euler  FilterMethod=Forward Euler  ControllerParametersSource=internal  P=Kp_Pitch  I=1  UseKiTs=off  D=Kd_Pitch  UseExternalDerivativeSource=off  N=N_Pitch  UseFilter=on  TunerSelectOption=Transfer Function Based (PID Tuner App)  InitialConditionSource=internal  InitialConditionForIntegrator=0  InitialConditionForFilter=0  DifferentiatorICPrevScaledInput=0  ExternalReset=none  TrackingMode=off  Kt=1  LimitOutput=off  SatLimitsSource=internal  UpperSaturationLimit=inf  LowerSaturationLimit=-inf  LinearizeAsGain=on  AntiWindupMode=none  Kb=1  LimitIntegrator=off  UpperIntegratorSaturationLimit=inf  LowerIntegratorSaturationLimit=-inf  POutMin=[]  POutMax=[]  IOutMin=[]  IOutMax=[]  DOutMin=[]  DOutMax=[]  NOutMin=[]  NOutMax=[]  SumOutMin=[]  SumOutMax=[]  SaturationOutMin=[]  SaturationOutMax=[]  PParamMin=[]  PParamMax=[]  IParamMin=[]  IParamMax=[]  DParamMin=[]  DParamMax=[]  NParamMin=[]  NParamMax=[]  KbParamMin=[]  KbParamMax=[]  KtParamMin=[]  KtParamMax=[]  KbOutMin=[]  KbOutMax=[]  KtOutMin=[]  KtOutMax=[]  IntegratorOutMin=[]  IntegratorOutMax=[]  FilterOutMin=[]  FilterOutMax=[]  SumI1OutMin=[]  SumI1OutMax=[]  SumI2OutMin=[]  SumI2OutMax=[]  SumI3OutMin=[]  SumI3OutMax=[]  SumI4OutMin=[]  SumI4OutMax=[]  SumDOutMin=[]  SumDOutMax=[]  DifferentiatorOutMin=[]  DifferentiatorOutMax=[]  FilterDiffOutCoefMin=[]  FilterDiffOutCoefMax=[]  ReciprocalOutMin=[]  ReciprocalOutMax=[]  SumDenOutMin=[]  SumDenOutMax=[]  SumNumOutMin=[]  SumNumOutMax=[]  DivideOutMin=[]  DivideOutMax=[]  UdiffTsProdOutMin=[]  UdiffTsProdOutMax=[]  NTsProdOutMin=[]  NTsProdOutMax=[]  UintegralTsProdOutMin=[]  UintegralTsProdOutMax=[]  UngainTsProdOutMin=[]  UngainTsProdOutMax=[]  ClampingZeroOutDataTypeStr=Inherit: Inherit via back propagation  ClampingZeroOutMin=[]  ClampingZeroOutMax=[]  FilterDenConstantOutDataTypeStr=Inherit: Inherit via back propagation  FilterDenConstantOutMin=[]  FilterDenConstantOutMax=[]  PCopyOutDataTypeStr=Inherit: Inherit via back propagation  PCopyOutMin=[]  PCopyOutMax=[]  NCopyOutDataTypeStr=Inherit: Inherit via back propagation  NCopyOutMin=[]  NCopyOutMax=[]  IntegratorContinuousStateAttributes=''  IntegratorStateMustResolveToSignalObject=off  IntegratorRTWStateStorageClass=Auto  FilterContinuousStateAttributes=''  FilterStateMustResolveToSignalObject=off  FilterRTWStateStorageClass=Auto  ParallelPVariant=InternalParameters  IdealPVariant=Disabled  IVariant=Disabled  DVariant=InternalParameters  IntegratorVariant=Disabled  SatVariant=Disabled  AWVariant=Disabled  PCopyVariant=Disabled  TRVariant=Disabled  FdbkBlocksVariant=Forward  IdealPFdbkVariant=Disabled  SatFdbkVariant=Disabled  DerivativeFilterVariant=ContFilter  NVariant=InternalParameters  NCopyVariant=Disabled  FilterICVariant=InternalICsFilter  IntegratorICVariant=Disabled  ExternalResetVariant=Disabled  TRSumVariant=Passthrough  SumFdbkVariant=Disabled  SumVariant=Sum_PD  TsampFilterVariant=InternalTs  TsampNgainVariant=Passthrough  TsampIntegralVariant=Disabled_SignalSpec  ExternalSaturationOutDataTypeStr=Inherit: Same as second input  DerivativeSourceVariant=ErrorSignal
  Sum : Sum  Inputs=|+-
  Sum1 : Sum  Inputs=|+-
  Sum2 : Sum  Inputs=|+-
  uPosition : Outport
  wires:
  Sum/1 -> Lateral_Position_PID/1
  xCmd/1 -> Sum/1
  x/1 -> Sum/2
  Lateral_Position_PID/1 -> Sum1/1
  Sum1/1 -> Pitch_PD_ Controller/1
  Theta/1 -> Sum1/2
  1_over_tau/1 -> Integrator/1
  Sum2/1 -> 1_over_tau/1
  Integrator/1 -> Sum2/2, uPosition/1
  Pitch_PD_ Controller/1 -> Sum2/1

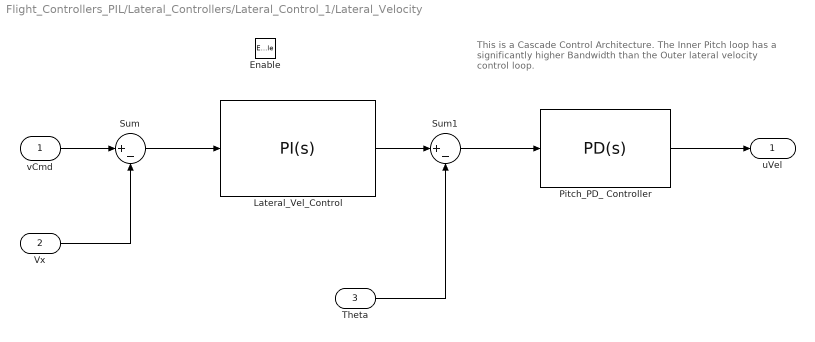
== system Flight_Controllers_PIL/Lateral_Controllers/Lateral_Control_1/Lateral_Velocity ==
  note: This is a Cascade Control Architecture.
      | The Inner Pitch loop has a significantly higher Bandwidth than
      | the Outer lateral velocity control loop.
  vCmd : Inport
  Vx : Inport  Port=2
  Theta : Inport  Port=3
  Enable : EnablePort
  Lateral_Vel_Control : slpidlib/PID Controller  Controller=PI  Form=Parallel  TimeDomain=Continuous-time  UseExternalTs=off  SampleTime=-1  IntegratorMethod=Forward Euler  FilterMethod=Forward Euler  ControllerParametersSource=internal  P=Kp_LatVel  I=Ki_LatVel  UseKiTs=off  D=0  UseExternalDerivativeSource=off  N=100  UseFilter=on  TunerSelectOption=Transfer Function Based (PID Tuner App)  InitialConditionSource=internal  InitialConditionForIntegrator=0  InitialConditionForFilter=0  DifferentiatorICPrevScaledInput=0  ExternalReset=none  TrackingMode=off  Kt=1  LimitOutput=off  SatLimitsSource=internal  UpperSaturationLimit=inf  LowerSaturationLimit=-inf  LinearizeAsGain=on  AntiWindupMode=none  Kb=1  LimitIntegrator=off  UpperIntegratorSaturationLimit=inf  LowerIntegratorSaturationLimit=-inf  POutMin=[]  POutMax=[]  IOutMin=[]  IOutMax=[]  DOutMin=[]  DOutMax=[]  NOutMin=[]  NOutMax=[]  SumOutMin=[]  SumOutMax=[]  SaturationOutMin=[]  SaturationOutMax=[]  PParamMin=[]  PParamMax=[]  IParamMin=[]  IParamMax=[]  DParamMin=[]  DParamMax=[]  NParamMin=[]  NParamMax=[]  KbParamMin=[]  KbParamMax=[]  KtParamMin=[]  KtParamMax=[]  KbOutMin=[]  KbOutMax=[]  KtOutMin=[]  KtOutMax=[]  IntegratorOutMin=[]  IntegratorOutMax=[]  FilterOutMin=[]  FilterOutMax=[]  SumI1OutMin=[]  SumI1OutMax=[]  SumI2OutMin=[]  SumI2OutMax=[]  SumI3OutMin=[]  SumI3OutMax=[]  SumI4OutMin=[]  SumI4OutMax=[]  SumDOutMin=[]  SumDOutMax=[]  DifferentiatorOutMin=[]  DifferentiatorOutMax=[]  FilterDiffOutCoefMin=[]  FilterDiffOutCoefMax=[]  ReciprocalOutMin=[]  ReciprocalOutMax=[]  SumDenOutMin=[]  SumDenOutMax=[]  SumNumOutMin=[]  SumNumOutMax=[]  DivideOutMin=[]  DivideOutMax=[]  UdiffTsProdOutMin=[]  UdiffTsProdOutMax=[]  NTsProdOutMin=[]  NTsProdOutMax=[]  UintegralTsProdOutMin=[]  UintegralTsProdOutMax=[]  UngainTsProdOutMin=[]  UngainTsProdOutMax=[]  ClampingZeroOutDataTypeStr=Inherit: Inherit via back propagation  ClampingZeroOutMin=[]  ClampingZeroOutMax=[]  FilterDenConstantOutDataTypeStr=Inherit: Inherit via back propagation  FilterDenConstantOutMin=[]  FilterDenConstantOutMax=[]  PCopyOutDataTypeStr=Inherit: Inherit via back propagation  PCopyOutMin=[]  PCopyOutMax=[]  NCopyOutDataTypeStr=Inherit: Inherit via back propagation  NCopyOutMin=[]  NCopyOutMax=[]  IntegratorContinuousStateAttributes=''  IntegratorStateMustResolveToSignalObject=off  IntegratorRTWStateStorageClass=Auto  FilterContinuousStateAttributes=''  FilterStateMustResolveToSignalObject=off  FilterRTWStateStorageClass=Auto  ParallelPVariant=InternalParameters  IdealPVariant=Disabled  IVariant=InternalParameters  DVariant=Disabled  IntegratorVariant=Continuous  SatVariant=Disabled  AWVariant=Passthrough  PCopyVariant=Disabled  TRVariant=Disabled  FdbkBlocksVariant=Forward  IdealPFdbkVariant=Disabled  SatFdbkVariant=Disabled  DerivativeFilterVariant=Disabled  NVariant=Disabled  NCopyVariant=Disabled_SignalSpec  FilterICVariant=Disabled  IntegratorICVariant=InternalICs  ExternalResetVariant=Disabled  TRSumVariant=Passthrough  SumFdbkVariant=Disabled  SumVariant=Sum_PI  TsampFilterVariant=InternalTs  TsampNgainVariant=Passthrough  TsampIntegralVariant=Disabled_SignalSpec  ExternalSaturationOutDataTypeStr=Inherit: Same as second input  DerivativeSourceVariant=Disabled
  Pitch_PD_ Controller : slpidlib/PID Controller  Controller=PD  Form=Parallel  TimeDomain=Continuous-time  UseExternalTs=off  SampleTime=-1  IntegratorMethod=Forward Euler  FilterMethod=Forward Euler  ControllerParametersSource=internal  P=Kp_Pitch  I=1  UseKiTs=off  D=Kd_Pitch  UseExternalDerivativeSource=off  N=N_Pitch  UseFilter=on  TunerSelectOption=Transfer Function Based (PID Tuner App)  InitialConditionSource=internal  InitialConditionForIntegrator=0  InitialConditionForFilter=0  DifferentiatorICPrevScaledInput=0  ExternalReset=none  TrackingMode=off  Kt=1  LimitOutput=off  SatLimitsSource=internal  UpperSaturationLimit=inf  LowerSaturationLimit=-inf  LinearizeAsGain=on  AntiWindupMode=none  Kb=1  LimitIntegrator=off  UpperIntegratorSaturationLimit=inf  LowerIntegratorSaturationLimit=-inf  POutMin=[]  POutMax=[]  IOutMin=[]  IOutMax=[]  DOutMin=[]  DOutMax=[]  NOutMin=[]  NOutMax=[]  SumOutMin=[]  SumOutMax=[]  SaturationOutMin=[]  SaturationOutMax=[]  PParamMin=[]  PParamMax=[]  IParamMin=[]  IParamMax=[]  DParamMin=[]  DParamMax=[]  NParamMin=[]  NParamMax=[]  KbParamMin=[]  KbParamMax=[]  KtParamMin=[]  KtParamMax=[]  KbOutMin=[]  KbOutMax=[]  KtOutMin=[]  KtOutMax=[]  IntegratorOutMin=[]  IntegratorOutMax=[]  FilterOutMin=[]  FilterOutMax=[]  SumI1OutMin=[]  SumI1OutMax=[]  SumI2OutMin=[]  SumI2OutMax=[]  SumI3OutMin=[]  SumI3OutMax=[]  SumI4OutMin=[]  SumI4OutMax=[]  SumDOutMin=[]  SumDOutMax=[]  DifferentiatorOutMin=[]  DifferentiatorOutMax=[]  FilterDiffOutCoefMin=[]  FilterDiffOutCoefMax=[]  ReciprocalOutMin=[]  ReciprocalOutMax=[]  SumDenOutMin=[]  SumDenOutMax=[]  SumNumOutMin=[]  SumNumOutMax=[]  DivideOutMin=[]  DivideOutMax=[]  UdiffTsProdOutMin=[]  UdiffTsProdOutMax=[]  NTsProdOutMin=[]  NTsProdOutMax=[]  UintegralTsProdOutMin=[]  UintegralTsProdOutMax=[]  UngainTsProdOutMin=[]  UngainTsProdOutMax=[]  ClampingZeroOutDataTypeStr=Inherit: Inherit via back propagation  ClampingZeroOutMin=[]  ClampingZeroOutMax=[]  FilterDenConstantOutDataTypeStr=Inherit: Inherit via back propagation  FilterDenConstantOutMin=[]  FilterDenConstantOutMax=[]  PCopyOutDataTypeStr=Inherit: Inherit via back propagation  PCopyOutMin=[]  PCopyOutMax=[]  NCopyOutDataTypeStr=Inherit: Inherit via back propagation  NCopyOutMin=[]  NCopyOutMax=[]  IntegratorContinuousStateAttributes=''  IntegratorStateMustResolveToSignalObject=off  IntegratorRTWStateStorageClass=Auto  FilterContinuousStateAttributes=''  FilterStateMustResolveToSignalObject=off  FilterRTWStateStorageClass=Auto  ParallelPVariant=InternalParameters  IdealPVariant=Disabled  IVariant=Disabled  DVariant=InternalParameters  IntegratorVariant=Disabled  SatVariant=Disabled  AWVariant=Disabled  PCopyVariant=Disabled  TRVariant=Disabled  FdbkBlocksVariant=Forward  IdealPFdbkVariant=Disabled  SatFdbkVariant=Disabled  DerivativeFilterVariant=ContFilter  NVariant=InternalParameters  NCopyVariant=Disabled  FilterICVariant=InternalICsFilter  IntegratorICVariant=Disabled  ExternalResetVariant=Disabled  TRSumVariant=Passthrough  SumFdbkVariant=Disabled  SumVariant=Sum_PD  TsampFilterVariant=InternalTs  TsampNgainVariant=Passthrough  TsampIntegralVariant=Disabled_SignalSpec  ExternalSaturationOutDataTypeStr=Inherit: Same as second input  DerivativeSourceVariant=ErrorSignal
  Sum : Sum  Inputs=|+-
  Sum1 : Sum  Inputs=|+-
  uVel : Outport
  wires:
  Sum/1 -> Lateral_Vel_Control/1
  Vx/1 -> Sum/2
  vCmd/1 -> Sum/1
  Pitch_PD_ Controller/1 -> uVel/1
  Theta/1 -> Sum1/2
  Lateral_Vel_Control/1 -> Sum1/1
  Sum1/1 -> Pitch_PD_ Controller/1

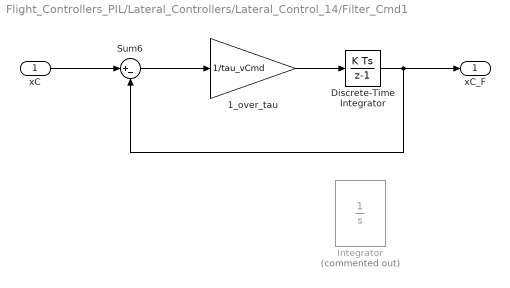
== system Flight_Controllers_PIL/Lateral_Controllers/Lateral_Control_14/Filter_Cmd1 ==
  xC : Inport  SampleTime=T
  1_over_tau : Gain  Gain=1/tau_vCmd
  Discrete-Time Integrator : DiscreteIntegrator  SampleTime=T  ICPrevOutput=DiscIntNeverNeededParam  ICPrevScaledInput=DiscIntNeverNeededParam
  Integrator : Integrator  Commented=on
  Sum6 : Sum  Inputs=|+-
  xC_F : Outport  SampleTime=T
  wires:
  Sum6/1 -> 1_over_tau/1
  xC/1 -> Sum6/1
  1_over_tau/1 -> Discrete-Time Integrator/1
  Discrete-Time Integrator/1 -> Sum6/2, xC_F/1

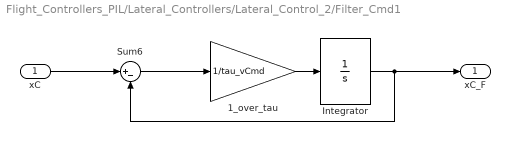
== system Flight_Controllers_PIL/Lateral_Controllers/Lateral_Control_2/Filter_Cmd1 ==
  xC : Inport
  1_over_tau : Gain  Gain=1/tau_vCmd
  Integrator : Integrator
  Sum6 : Sum  Inputs=|+-
  xC_F : Outport
  wires:
  Sum6/1 -> 1_over_tau/1
  xC/1 -> Sum6/1
  Integrator/1 -> xC_F/1, Sum6/2
  1_over_tau/1 -> Integrator/1

== system Flight_Controllers_PIL/Lateral_Controllers/Lateral_Control_3/Filter_Cmd1 ==
  xC : Inport
  1_over_tau : Gain  Gain=1/tau_xCmd
  Integrator : Integrator
  Sum6 : Sum  Inputs=|+-
  xC_F : Outport
  wires:
  Sum6/1 -> 1_over_tau/1
  xC/1 -> Sum6/1
  Integrator/1 -> xC_F/1, Sum6/2
  1_over_tau/1 -> Integrator/1

== system Flight_Controllers_PIL/Lateral_Controllers/Lateral_Control_4/Filter_Cmd1 ==
  xC : Inport
  1_over_tau : Gain  Gain=1/tau_vCmd
  Integrator : Integrator
  Sum6 : Sum  Inputs=|+-
  xC_F : Outport
  wires:
  Sum6/1 -> 1_over_tau/1
  xC/1 -> Sum6/1
  Integrator/1 -> xC_F/1, Sum6/2
  1_over_tau/1 -> Integrator/1

== matlab function Flight_Controllers_PIL/Vertical_Controller ==
  data: t input; fltSched input double; switchLines input; z_E input; zVel input; fireCmd output; Vertical_Mode output; Cntrl_telem output; m input; LandNowFl input
function [fireCmd, Vertical_Mode, Cntrl_telem] ... 
                                 = Control_Vert(t, fltSched, switchLines, z_E,zVel, m, LandNowFl)  
    %  Vertical Control Algotithm
    %    h is Altitude (m)
    %    hDot is Altitude Rate (m/s)
    %    hDot_Cmd is the Commanded Altitude Rate (m/s)
    %    m is the mass of the vehicle (kg)
    %    hyst_Width is the width of the hysteresis deadband (m/s)
    %          Will fire when vErr < -hyst_Width/2 and continue firing
    %          until vErr > hyst_Width/2.

validateattributes(t, {'double'}, {'scalar'})
validateattributes(LandNowFl, {'logical'}, {'scalar'})
% validateattributes(Xe, {'struct'}, {'scalar'})  % Bus becomes a Structure inside a Matlab function
% validateattributes(Vb, {'struct'}, {'scalar'})
% validateattributes(fltSched, {'numeric'}, {'column','numel',3})

% validateattributes(Xe, {'numeric'}, {'column','numel',3})  Used with Mux
%                                                       (NOT with a Bus)


velHyst = 0.20;  %   Hysteresis for the Vertical Velocity Phase Plane

persistent thr_previous
if isempty(thr_previous) 
    thr_previous = 0; % Initialize 
end

fireCmd = 0;

hErr = 0;   vErr = 0;


h = -1*z_E;  % m   "Z" position or the Altitude "h"
              %   Multiply by -1 because +Z is Down


hDot = -1*zVel;  % m/s   "Z" velocity or the Altitude rate "hDot"  (+Z is DOWN)



Vertical_Mode = interp1( fltSched(:,1), fltSched(:,2), t, 'previous');
vertCmd  = interp1( fltSched(:,1), fltSched(:,3), t, 'previous'); 

hCmd = 0;   hDot_Cmd = 0;

if Vertical_Mode == 1  % Mode 1 is Vertical Rate Control
    hDot_Cmd = vertCmd;
    hCmd = NaN;
    vErr = hDot - hDot_Cmd; % m/s  Velocity Error
    
    if vErr < -velHyst/2
        fireCmd = 1;
    elseif vErr > velHyst/2
        fireCmd = 0;
    else                           % You are in the Hysteresis Band
        if thr_previous > 0
            fireCmd = 1; % In the Hysteresis Band & Continue Firing
        else
            fireCmd = 0;  % Don't fire until you reach the bottom of the Hysteresis Band
        end
    end


elseif Vertical_Mode == 2   % Mode 2 is Vertical Postion Control (i.e. Hover)
    hCmd = vertCmd;
    hDot_Cmd = NaN;


   lowerSwitchLine = switchLines(  1: 4, :);  % See "run_AltitudePhasePlane_Design.m"
   lowerHystLine   = switchLines(  5:8, :);

   %% Find respective points on the upper & lower switch lines that correspond to hErr
   hErr = h - hCmd; % m/s  Altitude Error
   vErr = hDot - 0; % m/s  Velocity Error  (hDotCmd must = 0 for Postion Control)

   if hErr < lowerSwitchLine(1,1)  % In case h is outside the range of the PP design
       hErr = lowerSwitchLine(1,1);
   end
   if hErr > lowerSwitchLine(end,1)
       hErr = lowerSwitchLine(end,1);
end

%     formatSpec = '   t = %g  hErr = %g  vErr = %g';
%     str = sprintf(formatSpec, t, hErr, vErr)

hDot_err_lower = interpn( lowerSwitchLine(:,1), lowerSwitchLine(:,2), hErr );

hDot_err_lowerHyst = interpn( lowerHystLine(:,1), lowerHystLine(:,2), hErr );

%  Make Attitude Control Firing Decision   (Either Fire or don't and let gravity pull you down)
includeHysteresis = 1; %   Without hysteresis there is a risk you will rapidly pulse from
                       %      one side of a switch line to the other.
if includeHysteresis   %  ------------- With Hysteresis  -----------------
    
    if vErr < hDot_err_lower 
        fireCmd = 1;  % Fire the Center Cold Gas Engine
    
    elseif (vErr > hDot_err_lower) & (vErr < hDot_err_lowerHyst)
        fireCmd = thr_previous;  %   You are in the lower hysteresis band
   
    else fireCmd = 0;  % In the Drift zone
           fireCmd = 0;
    end

else  %    ----------------  No Hysteresis  -----------------------------
    if vErr < hDot_err_lower 
        fireCmd = 1;  % Fire
 
    else fireCmd = 0;  % In the Drift zone
    end
  end
end

% %  Display some data for debugging purposes.  Comment out when not needed.
% formatSpec = " Segment %2g  Prev Seg = %2g  t = %4g  t1 = %4g  t2 = %4g  VertVelCmd = %4g  VertPosCmd = %4g";
% str = sprintf(formatSpec, flightSegment, flightSegmentPrevious, t, t1, t2, VertVelCmd, VertPosCmd);
% disp(str)
%    formatSpec = "      LandNowFl = %2g ";
%    str = sprintf(formatSpec, single(LandNowFl) );
%    disp(str)


% Cntrl_telem = [t h hDot hDot_Cmd vErr thr_previous fireCmd];
Cntrl_telem = [t h hDot hDot_Cmd hCmd hErr vErr thr_previous fireCmd Vertical_Mode];

thr_previous = fireCmd;  % Set Previous Fire Command

== matlab function Flight_Controllers_PIL/Lateral_Controllers/Lateral_Control_3/Lateral_Flight_Plan ==
  data: xCmd output; t input; LatFlt_Schedule input
function xCmd  = Lateral_Schedule(t, LatFlt_Schedule)

%  For Controller version 3 there is only 1 Lateral Control Mode and that is
%    Position Control.  Velocity is "controlled" indirectly by how the
%    position command is structured.
%  The Lateral Flight Schedule is arranged as follows:
%        Column 1:  Time (sec)
%        Column 2:  Mode   Always Mode 2 for Position Control
%        Column 3:  xCmd   X Position Command
%        Column 4:  vLim   Currently NOT used

% validateattributes(t, {'double'}, {'scalar'})

xCmd  = interp1( LatFlt_Schedule(:,1), LatFlt_Schedule(:,3), t); 
% vLim  = interp1( LatFlt_Schedule(:,1), LatFlt_Schedule(:,4), t, 'previous'); 

% modeLat = 2; %  Always Postion Mode.  Keeping this so the plot script is 
             %     good for this and Control schemes with more than one
             %     mode.
